simulink model "MainSimu"  (R2020b)
settings: Solver=VariableStepAuto  StartTime=0.0  StopTime=10.0  RelTol=1e-3
settings Model: Creator=Aurelie  LastModifiedBy=Aurelie

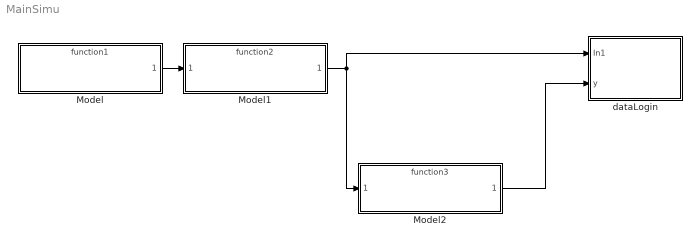
== system MainSimu ==
  Model : ModelReference  ModelNameDialog=function1  SimulationMode=Normal  ModelReferenceVersion=1.4
  Model1 : ModelReference  ModelNameDialog=function2  SimulationMode=Normal  ModelReferenceVersion=1.3
  Model2 : ModelReference  ModelNameDialog=function3  SimulationMode=Normal  ModelReferenceVersion=1.2
  dataLogin : Subsystem
  wires:
  Model/1 -> Model1/1
  Model1/1 -> Model2/1, dataLogin/1(In1)
  Model2/1 -> dataLogin/2(y)

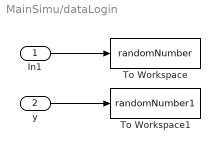
== system MainSimu/dataLogin ==
  In1 : Inport
  y : Inport  Port=2
  To Workspace : ToWorkspace  VariableName=randomNumber  SaveFormat=Timeseries  SampleTime=-1
  To Workspace1 : ToWorkspace  VariableName=randomNumber1  SaveFormat=Timeseries  SampleTime=-1
  wires:
  In1/1 -> To Workspace/1
  y/1 -> To Workspace1/1
